simulink model "sensorExpoler"  (R2026a)
settings: Solver=FixedStepDiscrete  StopTime=inf  FixedStep=0.001
undefined symbols (not defined in the file): Blocking, Non
libraries: eeGeneralControl x3, fl_lib x3, nesl_utility x3, amg_usbconverter_n_connect_lib x2, ee_lib x1, simulink x1
settings Model: Creator=pboon  LastModifiedBy=Lenovo

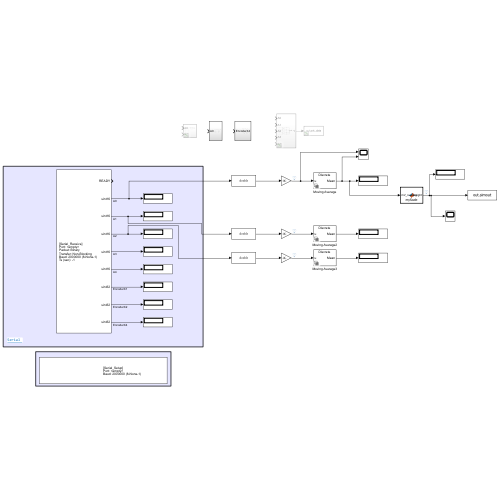
[thumbnail: Simulink's stored preview of the top-level diagram]
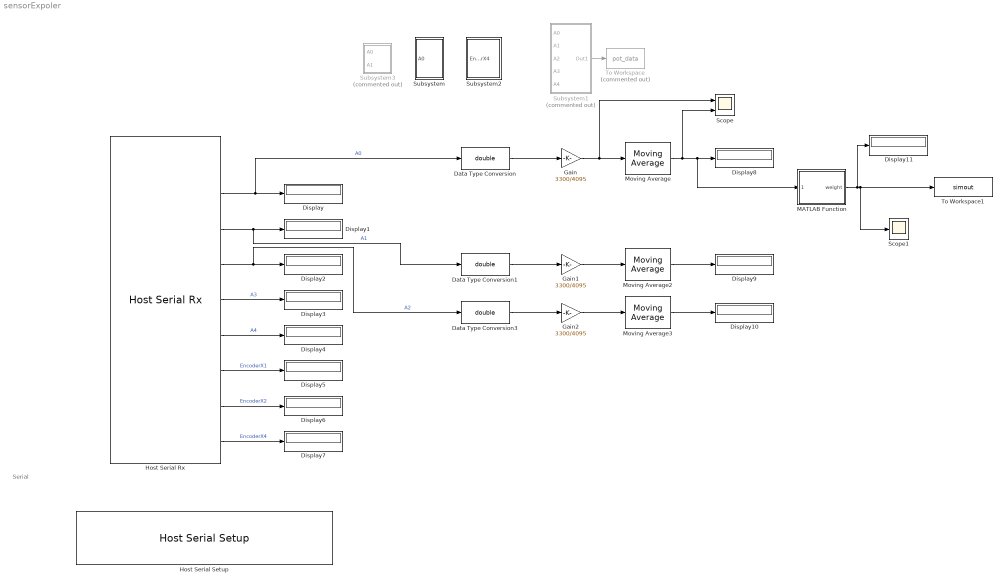
== system sensorExpoler ==
  note: Serial
  Data Type Conversion : DataTypeConversion  OutDataTypeStr=double  SaturateOnIntegerOverflow=off  RndMeth=Floor
  Data Type Conversion1 : DataTypeConversion  OutDataTypeStr=double  SaturateOnIntegerOverflow=off  RndMeth=Floor
  Data Type Conversion3 : DataTypeConversion  OutDataTypeStr=double  SaturateOnIntegerOverflow=off  RndMeth=Floor
  Display{,1..11} (12 alike) : Display
  Gain : Gain  Gain=3300/4095
  Gain1 : Gain  Gain=3300/4095
  Gain2 : Gain  Gain=3300/4095
  Host Serial Rx : amg_usbconverter_n_connect_lib/Host Serial Rx  conf=rx  port=<auto>  baudrate=2000000  databits=8  parity=None  stopbit=1  flowcontrol=None  transfer=Non-Blocking  timeout=5  packetmode=Binary  enableinitialvalues=off  initialvalues=[]  binheader='25'  binterminator='4E 4E'  porttype_double=0  porttype_single=0  porttype_int8=0  porttype_uint8=0  porttype_int16=0  porttype_uint16=5  porttype_int32=0  porttype_uint32=3  asciiformat='%d,%f'  rx_asciiterminator="CRLF (0x0D 0x0A - \"\\r\\n\")"  tx_asciiterminator="CRLF (0x0D 0x0A - \"\\r\\n\")"  sampletime=0.001  enablecustomportlabel=off  cinputportlabel=0  coutputportlabel=A  portpinstr=0  blockid=HostSerialRx  inputporttype=[]  inputportwidth=[]  inputportlabel={}  outputporttype=[3 5 5 5 5 5 7 7 7]  outputportwidth=[1 1 1 1 1 1 1 1 1]  outputportlabel={'READY','uint16','uint16','uint16','uint16','uint16','uint32','uint32','uint32'}  compat=0  optionstring=[]  autoport='<empty>'
  Host Serial Setup : amg_usbconverter_n_connect_lib/Host Serial Setup  conf=setup  port=<auto>  baudrate=2000000  databits=8  parity=None  stopbit=1  flowcontrol=None  transfer=Blocking  timeout=2  packetmode=Binary  initialvalues=[]  binheader='7E 7E'  binterminator='03 03'  porttype_double=0  porttype_single=1  porttype_int8=0  porttype_uint8=0  porttype_int16=0  porttype_uint16=0  porttype_int32=0  porttype_uint32=2  asciiformat='%d %u %x'  rx_asciiterminator="CRLF (0x0D 0x0A - \"\\r\\n\")"  tx_asciiterminator="CRLF (0x0D 0x0A - \"\\r\\n\")"  sampletime=-1  enablecustomportlabel=off  cinputportlabel=0  coutputportlabel=A  portpinstr=0  blockid=HostSerialSetup  inputporttype=[]  inputportwidth=[]  inputportlabel={}  outputporttype=[]  outputportwidth=[]  outputportlabel={}  compat=0  optionstring=[]  autoport='<empty>'
  MATLAB Function : MATLAB Function  TreatAsAtomicUnit=on
  Moving Average : eeGeneralControl/Moving Average  VariantControl=Variant1  LabelModeActiveChoice=Discrete  f=2.7862  x0=0  BufferSize=8192  Ts=-1
      settings: LibrarySourceBlock=ee_sl_lib/General Control/Moving Average
  Moving Average2 : eeGeneralControl/Moving Average  VariantControl=Variant1  LabelModeActiveChoice=Discrete  f=2.7862  x0=0  BufferSize=8192  Ts=-1
      settings: LibrarySourceBlock=ee_sl_lib/General Control/Moving Average
  Moving Average3 : eeGeneralControl/Moving Average  VariantControl=Variant1  LabelModeActiveChoice=Discrete  f=2.7862  x0=0  BufferSize=8192  Ts=-1
      settings: LibrarySourceBlock=ee_sl_lib/General Control/Moving Average
  Scope : Scope  NumInputPorts=2
      settings: DataLoggingVariableName=ScopeData3
  Scope1 : Scope
      settings: DataLoggingVariableName=ScopeData4
  Subsystem : Subsystem
  Subsystem1 : Subsystem  Commented=on
  Subsystem2 : Subsystem
  Subsystem3 : Subsystem  Commented=on
  To Workspace : ToWorkspace  Commented=on  VariableName=pot_data  SampleTime=-1
  To Workspace1 : ToWorkspace  VariableName=simout  SaveFormat=Timeseries  SampleTime=-1
  wires:
  Host Serial Rx/2 -> Data Type Conversion/1, Display/1  "A0"
  Host Serial Rx/4 -> Data Type Conversion3/1, Display2/1  "A2"
  Host Serial Rx/6 -> Display4/1  "A4"
  Host Serial Rx/8 -> Display6/1  "EncoderX2"
  Host Serial Rx/3 -> Data Type Conversion1/1, Display1/1  "A1"
  Host Serial Rx/5 -> Display3/1  "A3"
  Host Serial Rx/7 -> Display5/1  "EncoderX1"
  Host Serial Rx/9 -> Display7/1  "EncoderX4"
  Subsystem1/1(Out1) -> To Workspace/1
  Data Type Conversion/1 -> Gain/1
  Data Type Conversion1/1 -> Gain1/1
  Data Type Conversion3/1 -> Gain2/1
  Gain/1 -> Scope/1, Moving Average/1
  Moving Average/1 -> Scope/2, MATLAB Function/1(mV_reading), Display8/1
  Moving Average2/1 -> Display9/1
  Gain1/1 -> Moving Average2/1
  Gain2/1 -> Moving Average3/1
  Moving Average3/1 -> Display10/1
  MATLAB Function/1(weight) -> To Workspace1/1, Scope1/1, Display11/1

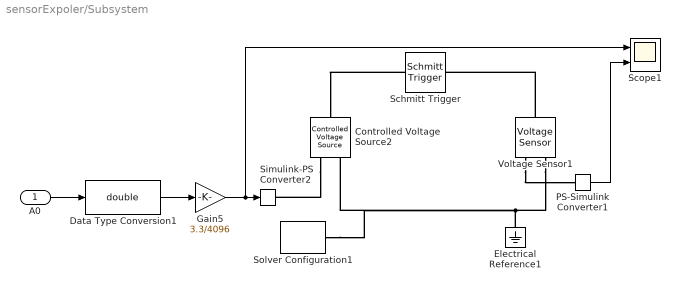
== system sensorExpoler/Subsystem ==
  A0 : Inport
  Controlled Voltage Source2 : fl_lib/Electrical/Electrical Sources/Controlled Voltage Source
  Data Type Conversion1 : DataTypeConversion  OutDataTypeStr=double  SaturateOnIntegerOverflow=off  RndMeth=Floor
  Electrical Reference1 : fl_lib/Electrical/Electrical Elements/Electrical Reference
  Gain5 : Gain  Gain=3.3/4096
  PS-Simulink Converter1 : nesl_utility/PS-Simulink Converter  PhysicalDomain=network_engine_domain  SubClassName=ps_output  LeftPortType=input  RightPortType=output  PseudoPeriodic=off  Frequencies=[]  VectorFormat=inherit  Unit=inherit  AffineConversion=off
  Schmitt Trigger : ee_lib/Integrated Circuits/Logic/Schmitt Trigger  V_IL=1.2 V  V_IH=2 V  C_IN=5 pF  output_type=ee.enum.ic.outputType.linear  V_OL=0 V  V_OH=3.3 V  V_CC=5 V  V_meas=5 V  R_OUT=25 Ohm  R_OH=[25, 250] Ohm  I_OH=63 mA  R_OL=[30, 800] Ohm  I_OL=-45 mA  Delay=25 ns  Ron=5 Ohm  Vf=0.6 V  output_state=ee.enum.ic.initialState.low
  Scope1 : Scope  NumInputPorts=2
      settings: ActiveDisplayYMinimum=0.97696838378906259  ActiveDisplayYMaximum=3.5581146240234376
  Simulink-PS Converter2 : nesl_utility/Simulink-PS Converter  PhysicalDomain=network_engine_domain  SubClassName=ps_input  LeftPortType=input  RightPortType=output  PseudoPeriodic=off  Frequencies=[]  NoiseDistribution=none  NoiseParameters=[]  Unit=1  AffineConversion=off  FilteringAndDerivatives=provide  SimscapeFilterOrder=1  InputFilterTimeConstant=0.001  UdotUserProvided=0
  Solver Configuration1 : nesl_utility/Solver Configuration  PhysicalDomain=network_engine_domain  SubClassName=solver  LeftPortType=input  RightPortType=generic  Tones=[]  Harmonics=[]  SimulateNoise=off  Profile=off  UseLocalSampling=off  EnableSwitchedLinearOptims=on  FrequencyDomain=off  UseCCode=off  RelTol=0.001  AbsTol=0.001  MinStep=1e-09  ToWorkspace=off  RevertToSquareIcSolve=off  NumHomotopyIterations=100  PhasorMode=off  PhasorModeNumHarmonics=1  ConsistencySolver=NEWTON_XTOL_AFTER_FTOL  CanonicalOrdering=CANONICAL  OptimizeIntermediates=OPTIMIZED  IndexReductionMethod=DerivativeReplacement  DoDC=on  ResidualTolerance=1e-09  ConsistencyTolSource=GLOBAL  ConsistencyAbsTol=0.001  ConsistencyRelTol=0.001  ConsistencyTolFactor=0.001  UseLocalSolver=on  LocalSolverChoice=NE_BACKWARD_EULER_ADVANCER  ResolveIndetEquations=on  FunctionEvalNumThread=1  LocalSolverSampleTime=0.001  DoFixedCost=off  MaxNonlinIter=3  MaxModeIter=2  ComputeImpulses=off  ImpulseIterations=2  LinearAlgebra=auto  LinearAlgebraNumThread=0  EquationFormulation=NE_TIME_EF  DelaysMemoryBudget=1024  AutomaticFiltering=on  FilteringTimeConstant=0.001  PartitionStorageMethod=AS_NEEDED  PartitionMemoryBudget=1024  PartitionMethod=ROBUST  MultibodyUseLocalSolver=off  MultibodyLocalSolverChoice=ODE1  MultibodyLocalSolverSampleTime=0.001
  Voltage Sensor1 : fl_lib/Electrical/Electrical Sensors/Voltage Sensor
  wires:
  PS-Simulink Converter1/1 -> Scope1/2
  Data Type Conversion1/1 -> Gain5/1
  A0/1 -> Data Type Conversion1/1
  Gain5/1 -> Scope1/1, Simulink-PS Converter2/1
  connections:
  Voltage Sensor1/RConn1 -- PS-Simulink Converter1/LConn1
  Voltage Sensor1/LConn1 -- Schmitt Trigger/RConn1
  Controlled Voltage Source2/RConn1 -- Simulink-PS Converter2/RConn1
  Schmitt Trigger/LConn1 -- Controlled Voltage Source2/LConn1
  Voltage Sensor1/RConn2 -- Controlled Voltage Source2/RConn2 -- Solver Configuration1/RConn1 -- Electrical Reference1/LConn1

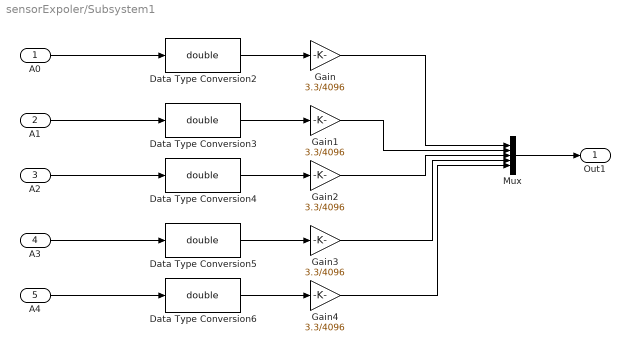
== system sensorExpoler/Subsystem1 ==
  A0 : Inport
  A1 : Inport  Port=2
  A2 : Inport  Port=3
  A3 : Inport  Port=4
  A4 : Inport  Port=5
  Data Type Conversion{2..6} (5 alike) : DataTypeConversion  OutDataTypeStr=double  SaturateOnIntegerOverflow=off  RndMeth=Floor
  Gain{,1..4} (5 alike) : Gain  Gain=3.3/4096
  Mux : Mux  Inputs=5
  Out1 : Outport
  wires:
  Data Type Conversion5/1 -> Gain3/1
  A3/1 -> Data Type Conversion5/1
  Gain2/1 -> Mux/3
  Data Type Conversion4/1 -> Gain2/1
  Gain1/1 -> Mux/2
  A2/1 -> Data Type Conversion4/1
  Data Type Conversion3/1 -> Gain1/1
  Data Type Conversion6/1 -> Gain4/1
  Gain/1 -> Mux/1
  Data Type Conversion2/1 -> Gain/1
  Gain4/1 -> Mux/5
  Gain3/1 -> Mux/4
  A4/1 -> Data Type Conversion6/1
  A0/1 -> Data Type Conversion2/1
  Mux/1 -> Out1/1
  A1/1 -> Data Type Conversion3/1

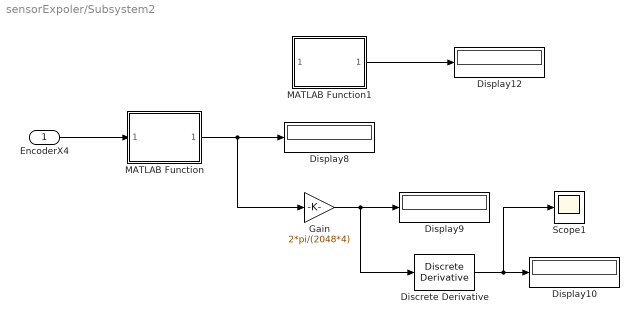
== system sensorExpoler/Subsystem2 ==
  EncoderX4 : Inport
  Discrete Derivative : simulink/Discrete/Discrete Derivative  gainval=1.0  ICPrevScaledInput=0.0  OutMin=[]  OutMax=[]  OutDataTypeStr=double  OutputDataTypeScalingMode=double  OutDataType=fixdt(1, 16)  OutScaling=2^-10  DoSatur=off
  Display{8..10,12} (4 alike) : Display
  Gain : Gain  Gain=2*pi/(2048*4)
  MATLAB Function : MATLAB Function  TreatAsAtomicUnit=on
  MATLAB Function1 : MATLAB Function  TreatAsAtomicUnit=on
  Scope1 : Scope
      settings: ActiveDisplayYMinimum=-1038.9353790526959  ActiveDisplayYMaximum=1860.6673564583091  DataLoggingVariableName=ScopeData2
  wires:
  Discrete Derivative/1 -> Scope1/1, Display10/1
  MATLAB Function1/1(angle_rad) -> Display12/1
  MATLAB Function/1(unwrapped_count) -> Gain/1, Display8/1
  Gain/1 -> Discrete Derivative/1, Display9/1
  EncoderX4/1 -> MATLAB Function/1(current_count)

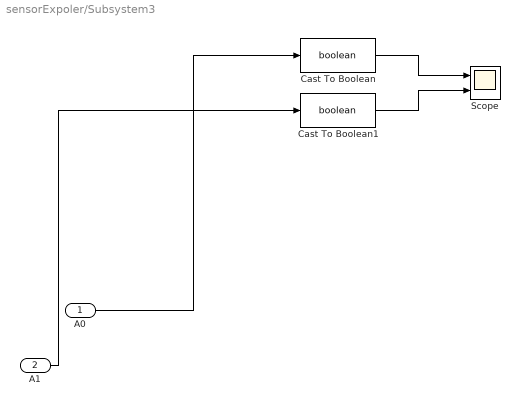
== system sensorExpoler/Subsystem3 ==
  A0 : Inport
  A1 : Inport  Port=2
  Cast To Boolean : DataTypeConversion  OutDataTypeStr=boolean  SaturateOnIntegerOverflow=off  RndMeth=Floor
  Cast To Boolean1 : DataTypeConversion  OutDataTypeStr=boolean  SaturateOnIntegerOverflow=off  RndMeth=Floor
  Scope : Scope  NumInputPorts=2
  wires:
  Cast To Boolean1/1 -> Scope/2
  A0/1 -> Cast To Boolean/1
  A1/1 -> Cast To Boolean1/1
  Cast To Boolean/1 -> Scope/1

== matlab function sensorExpoler/Subsystem2/MATLAB Function ==
  data: current_count input; unwrapped_count output
function unwrapped_count = WrapAround(current_count)
    current_count = double(current_count);

    ARR = 65535; 
    
    max_counts = ARR + 1;
    half_counts = max_counts / 2;
    
    persistent prev_count total_count
    if isempty(prev_count)
        prev_count = current_count;
        total_count = 0.0;
    end
    
    delta = current_count - prev_count;
    
    if delta < -half_counts
        delta = delta + max_counts;
    elseif delta > half_counts
        delta = delta - max_counts;
    end
    
    total_count = total_count + delta;
    prev_count = current_count;
    
    unwrapped_count = total_count;
end

== matlab function sensorExpoler/MATLAB Function ==
  data: mV_reading input; weight output
function weight = myScale(mV_reading)
    weight = (mV_reading - 27.47212038) / 0.2326;
end

== matlab function sensorExpoler/Subsystem2/MATLAB Function1 ==
  data: current_count input; angle_rad output
function angle_rad = EncoderHomingAngle(current_count)
    ARR = 65535;                 % ค่า Counter Period ของ Timer ใน STM32
    timer_max = ARR + 1;
    half_timer = timer_max / 2;  
    
    CPR = 8192;   % Counts Per Revolution)              
    
    persistent prev_count;
    persistent total_count;

    if isempty(prev_count)
        prev_count = current_count;
        total_count = 0;
    end

    delta = current_count - prev_count;

    if delta < -half_timer
        delta = delta + timer_max;
    elseif delta > half_timer
        delta = delta - timer_max;
    end

    total_count = total_count + delta;

    count_in_rev = mod(total_count, CPR);

    angle_rad = (count_in_rev / CPR) * (2 * pi);
    prev_count = current_count;
end
